simulink model "AaDdCc"  (R2024a)
settings: Solver=VariableStepAuto  StartTime=0.0  StopTime=5  RelTol=1e-3
libraries: dspvision x1, dspsigops x1
settings Model: Creator=User
settings RTWCC: GPUComputeCapability=3.5

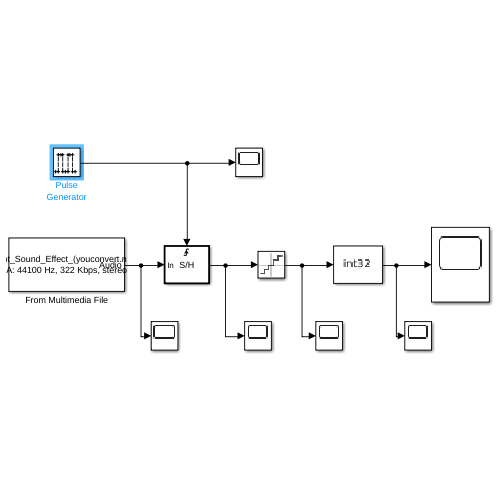
[thumbnail: Simulink's stored preview of the top-level diagram]
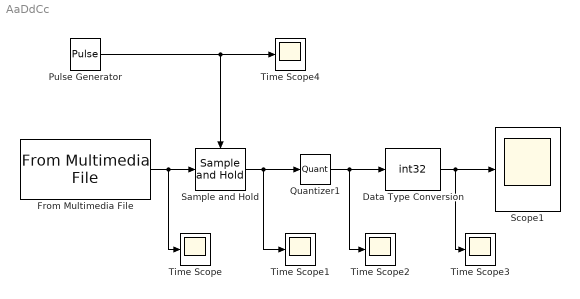
== system AaDdCc ==
  Data Type Conversion : DataTypeConversion  OutDataTypeStr=int32  SaturateOnIntegerOverflow=off  RndMeth=Floor
  From Multimedia File : dspvision/From Multimedia File  inputFilename=/MATLAB Drive/GUNSHOT SOUND FILE/Gunshot_Sound_Effect_(youconvert.net).mp3  readRange=[1 Inf]  loop=on  numPlays=inf  outputStreams=Audio only  videoDataType=single  audioDataType=double  inheritSampleTime=on  userDefinedSampleTime=1/30  noAudioOutput=off  isIntensityVideo=off  fourcc=RGB  colorVideoFormat=Separate color signals  outputEOF=off  dataOrg=Column-major  audioFrameSize=1024  computeAudioFrameSize=off  outSamplingMode=Sample based
      settings: LibrarySourceBlock=dspsrcs4/From Multimedia File
  Pulse Generator : DiscretePulseGenerator  Period=100  PulseWidth=50  SampleTime=0.00005
  Quantizer1 : Quantizer  QuantizationInterval=0.25
  Sample and Hold : dspsigops/Sample and Hold  trig=Rising edge  initCond=0  latchinput=off
  Scope1 : Scope
  Time Scope{,1..4} (5 alike) : Scope
  wires:
  Pulse Generator/1 -> Time Scope4/1, Sample and Hold/Trigger
  From Multimedia File/1 -> Time Scope/1, Sample and Hold/1
  Sample and Hold/1 -> Time Scope1/1, Quantizer1/1
  Data Type Conversion/1 -> Time Scope3/1, Scope1/1
  Quantizer1/1 -> Time Scope2/1, Data Type Conversion/1
